simulink model "fenxi_3kuangtu"  (R2020b)
settings: Solver=VariableStepAuto  StartTime=0.0  StopTime=200  RelTol=1e-3
settings Model: Creator=19017  LastModifiedBy=19017

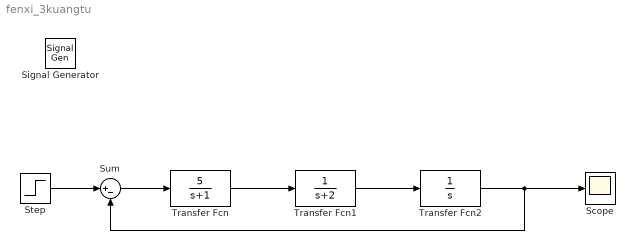
== system fenxi_3kuangtu ==
  Scope : Scope
  Signal Generator : SignalGenerator  Units=rad/sec
  Step : Step  SampleTime=0
  Sum : Sum  Inputs=|+-
  Transfer Fcn : TransferFcn  Numerator=[5]  Denominator=[1 1]
  Transfer Fcn1 : TransferFcn  Denominator=[1 2]
  Transfer Fcn2 : TransferFcn  Denominator=[1 0]
  wires:
  Transfer Fcn1/1 -> Transfer Fcn2/1
  Transfer Fcn/1 -> Transfer Fcn1/1
  Sum/1 -> Transfer Fcn/1
  Transfer Fcn2/1 -> Scope/1, Sum/2
  Step/1 -> Sum/1
